simulink model "CM"  (R2017a)
settings: Solver=VariableStepAuto  StartTime=0.0  StopTime=10  FixedStep=0.01  RelTol=1e-3
values from neighbouring files (symbols this model uses):
  alpha = 0.780    (= 0.78)    [CompartmentalModel.m]
  beta = 0.208    [CompartmentalModel.m]
  delta = 2.92    [CompartmentalModel.m]
  gamma = 4.34    [CompartmentalModel.m]
settings Model: Creator=Jake Tweedle  LastModifiedBy=Jake Tweedle

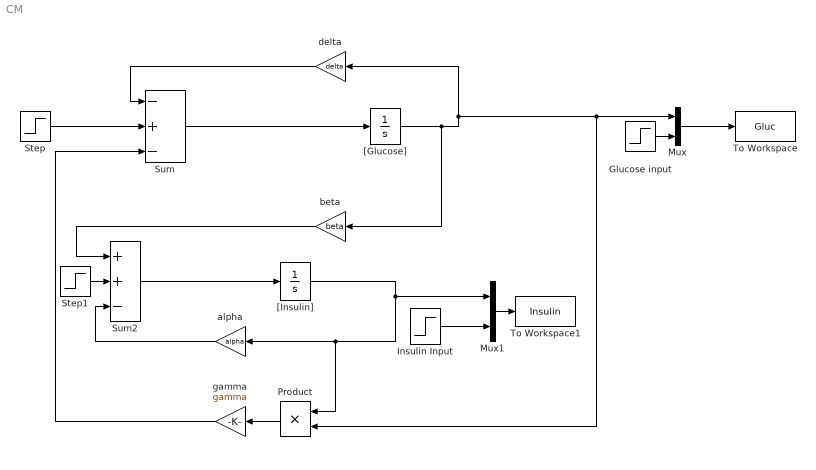
== system CM ==
  Glucose input : Step  After=0  SampleTime=0
  Insulin Input : Step  After=70  SampleTime=0
  Mux : Mux  Inputs=2
  Mux1 : Mux  Inputs=2
  Product : Product
  Step : Step  After=0  SampleTime=0
  Step1 : Step  After=70  SampleTime=0
  Sum : Sum  Inputs=-||+||-
  Sum2 : Sum  Inputs=+||+||-
  To Workspace : ToWorkspace  VariableName=Gluc  SaveFormat=Timeseries  SampleTime=-1
  To Workspace1 : ToWorkspace  VariableName=Insulin  SaveFormat=Timeseries  SampleTime=-1
  "[Glucose]" : Integrator
  "[Insulin]" : Integrator
  alpha : Gain  Gain=alpha
  beta : Gain  Gain=beta
  delta : Gain  Gain=delta
  gamma : Gain  Gain=gamma
  wires:
  Sum2/1 -> "[Insulin]"/1
  "[Glucose]"/1 -> Product/2, Mux/1, delta/1, beta/1
  Sum/1 -> "[Glucose]"/1
  gamma/1 -> Sum/3
  delta/1 -> Sum/1
  Step1/1 -> Sum2/2
  alpha/1 -> Sum2/3
  Step/1 -> Sum/2
  beta/1 -> Sum2/1
  Insulin Input/1 -> Mux1/2
  Glucose input/1 -> Mux/2
  Mux/1 -> To Workspace/1
  Mux1/1 -> To Workspace1/1
  "[Insulin]"/1 -> Mux1/1, Product/1, alpha/1
  Product/1 -> gamma/1
